simulink library "Lib_PF_BusLoadDC_TMATS"  (R2020b)
settings: Solver=ode45  StartTime=0.0  StopTime=10.0  RelTol=1e-3  EnableMultiTasking=on
Description:
  | Thomas Modules
settings Model: Creator=jwchapm2  LastModifiedBy=mebell
settings DataIOCC: LimitDataPoints=on  SaveFormat=Array  ReturnWorkspaceOutputs=off
settings OptimizationCC: ExpressionDepthLimit=2147483647  LifeSpan=inf
settings DebuggingCC: UnderspecifiedInitializationDetection=Classic  MergeDetectMultiDrivingBlocksExec=none  SolverPrmCheckMsg=warning  StateNameClashWarn=warning  SFUnexpectedBacktrackingDiag=warning  SFNoUnconditionalDefaultTransitionDiag=warning  SFExecutionAtInitializationDiag=none  ArithmeticOperatorsInVariantConditions=warning
settings HardwareCC: ProdBitPerPointer=32  ProdBitPerSizeT=32  ProdBitPerPtrDiffT=32  ProdLargestAtomicFloat=None  ProdIntDivRoundTo=Undefined  ProdEndianess=Unspecified  ProdWordSize=32  ProdHWDeviceType=32-bit Generic
settings ModelReferenceCC: PropagateSignalLabelsOutOfModel=off
settings SFSimCC: SimUseLocalCustomCode=off  CustomCodeUndefinedFunction=UseInterfaceOnly
settings RTWCC: RTWUseLocalCustomCode=off
settings CodeAppCC: StateflowObjectComments=on
settings GRTTargetCC: TargetLangStandard=C89/C90 (ANSI)
settings ConfigComp: CovMetricSettings=dw  CovSaveCumulativeToWorkspaceVar=on  CovSaveSingleToWorkspaceVar=on  CovExternalEMLEnable=off

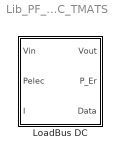
== system Lib_PF_BusLoadDC_TMATS ==
  LoadBus DC : Subsystem  mask{P_M=2, BlkNm_M=double(gcb)}
      mask prompts: P_M "P_M - Real power"; BlkNm_M "Block name as double for simulink output"

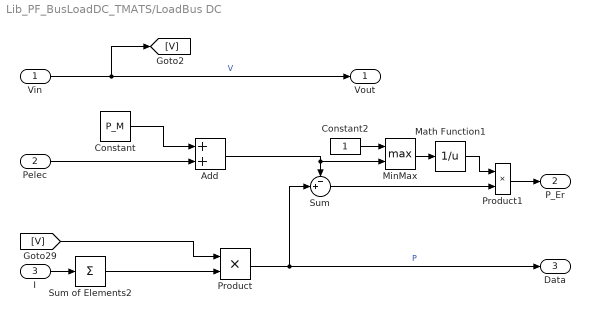
== system Lib_PF_BusLoadDC_TMATS/LoadBus DC ==
  Vin : Inport
  Pelec : Inport  Port=2
  I : Inport  Port=3
  Add : Sum
  Constant : Constant  Value=P_M
  Constant2 : Constant
  Math Function1 : Math  Operator=reciprocal  SignedPower=on  SaturateOnIntegerOverflow=on
  MinMax : MinMax  Function=max  Inputs=2
  Product : Product
  Product1 : Product
  Sum : Sum  Inputs=-+|
  Sum of Elements2 : Sum  Inputs=+
  Vout : Outport
  P_Er : Outport  Port=2
  Data : Outport  Port=3
  wires:
  Sum of Elements2/1 -> Product/2
  [V] -> Product/1
  I/1 -> Sum of Elements2/1
  Product/1 -> Data/1, Sum/2  "P"
  Vin/1 -> Vout/1, [V]  "V"
  Pelec/1 -> Add/2
  Constant2/1 -> MinMax/1
  MinMax/1 -> Math Function1/1
  Math Function1/1 -> Product1/1
  Product1/1 -> P_Er/1
  Sum/1 -> Product1/2
  Constant/1 -> Add/1
  Add/1 -> MinMax/2, Sum/1
